simulink library "allblocks_alteradspbuilder2"  (Simulink 7.6)
(part 3 of 4)

      mask Help: helpview(char(com.altera.dspbuilder.simulation.Cache.getBlockTemplate('BlockFactory', 'com.altera.dspbuilder.blockset.arithmetic.SumOfProducts').getHelpFile))
      mask StyleString: popup(Signed Integer|Unsigned Integer|Signed Fractional|Unsigned Fractional),edit,edit,edit,edit,edit,edit,edit,edit,checkbox,edit,edit,edit,popup(Distributed Arithmetic|Dedicated Multiplier Circuitry|Auto),checkbox,checkbox
      mask CallbackString: |||||||||alt_dspbuilder_update_gui('BlockFactory', 'com.altera.dspbuilder.blockset.arithmetic.SumOfProducts', 'full_resolution', 9);||||||
      mask TabNameString: Main,Main,Main,Main,Main,Main,Main,Main,Main,Optional Port Sizing,Optional Port Sizing,Optional Port Sizing,Optional Port Sizing,Optional Ports and Settings,Optional Ports and Settings,Optional Ports and Settings
      mask Display:
      | port_label('input', 1, 'a0');
      | port_label('input', 2, 'a1');
      | port_label('input', 3, 'a2');
      | port_label('input', 4, 'a3');
      | port_label('output', 1, 'q(17:0)');
      | plot([0.9 0.75 0.85 0.75 0.9], [0.15 0.15 0.1 0.05 0.05])
  TestBench : S-Function  LoadFcn=|  FunctionName=sTestBench  Parameters=enable advancedMode modelSimGui maxDisplayErrors mismatchErrorLevel simdatafile  EnableBusSupport=off  mask(TestBench AlteraBlockset){enable=on, advancedMode=off, modelSimGui=off, maxDisplayErrors=10, mismatchErrorLevel=Error, simdatafile=}
      | alt_dspbuilder_load_block(gcb, 'BlockFactory', 'com.altera.dspbuilder.blockset.altlab.TestBench');
      | alt_dspbuilder_init_testbench
      mask prompts: enable "Enable test bench generation"; advancedMode "Use advanced mode"; modelSimGui "Launch ModelSim in Graphical mode"; maxDisplayErrors "Maximum number of errors to display"; mismatchErrorLevel "Error level for mismatches"
      mask help:
      | Controls automatic generation of a test bench. Enabling testbench generation may slow simulation as all input and output values are stored to a file.
      |
      | If the ModelSim executable (vsim.exe) is available on your path, you can load the testbench into ModelSim and compare the results with Simulink. You can optionally launch the ModelSim GUI to visually view the ModelSim simulation.
      mask init:
      | alt_dspbuilder_init_testbench('BlockFactory', 'com.altera.dspbuilder.blockset.altlab.TestBench', { enable advancedMode modelSimGui maxDisplayErrors mismatchErrorLevel simdatafile });
      settings: CopyFcn=alt_dspbuilder_add_block(gcb, 'BlockFactory', 'com.altera.dspbuilder.blockset.altlab.TestBench');  UndoDeleteFcn=alt_dspbuilder_add_block(gcb, 'BlockFactory', 'com.altera.dspbuilder.blockset.altlab.TestBench');  NameChangeFcn=alt_dspbuilder_block_renamed(gcb);
      settings: DeleteFcn=|
      | alt_dspbuilder_internal_remove_testbench(gcb)
      | 
      | com.altera.dspbuilder.simulation.Mask.delete(gcb);
      settings: PostSaveFcn=|
      | alt_dspbuilder_block_saved(gcb);
      | alt_dspbuilder_init_testbench
      settings: OpenFcn=|
      | com.altera.dspbuilder.simulation.Mask.simpleInit('BlockFactory', 'com.altera.dspbuilder.blockset.altlab.TestBench', bdroot(gcb), gcb);
      | alt_testbenchLaunch(gcb)
      mask Help: helpview(char(com.altera.dspbuilder.simulation.Cache.getBlockTemplate('BlockFactory', 'com.altera.dspbuilder.blockset.altlab.TestBench').getHelpFile))
      mask Display: fprintf('TestBench\non');
  True Dual-Port RAM : S-Function  LoadFcn=alt_dspbuilder_load_block(gcb, 'BlockFactory', 'com.altera.dspbuilder.blockset.storage.TrueDualRam');  FunctionName=sGeneric  Parameters=numwords BusType bwl bwr memory_type ram_type dont_care initialization init_file init_array register_outputs use_ena ClockPhase pipeline_display allowFloatingPointOverride logOutputs logFile  EnableBusSupport=off  mask(True Dual-Port RAM AlteraBlockset){numwords=16, BusType=Signed Integer, bwl=8, bwr=0, memory_type=AUTO, ram_type=TrueDualRAM, dont_care=off, initialization=Blank, init_file=input.hex, init_array=[0:1:15], register_outputs=off, use_ena=off, ClockPhase=1, pipeline_display=1, allowFloatingPointOverride=on, logOutputs=off, logFile=D:\\allblocks%5Falteradspbuilder2_True+Dual-Port+RAM%3A%3Aq%5Fa.fixedpointlog,D:\\allblocks%5Falteradspbuilder2_True+Dual-Port+RAM%3A%3Aq%5Fb.fixedpointlog,}
      mask prompts: numwords "Number Of Words"; BusType "Data Type"; bwl "[Number Of Bits].[]"; bwr "[].[Number Of Bits]"; memory_type "Memory Block Type"; ram_type "RAM type"; dont_care "Use DONT_CARE when reading from and writing to the same address"; init_file "Input HEX File"; init_array "MATLAB Array"; register_outputs "Register Output Ports"; use_ena "Use Enable Port (ena)"; ClockPhase "Clock Phase Selection"; pipeline_display "Number Of Pipeline Stages (Calculated)"; allowFloatingPointOverride "Allow Floating Point Override For This Block"
      mask help:
      | Maps data to embedded RAM in Altera devices. Two read and two write ports allow true dual access.
      |
      | The True Dual-Port RAM block accepts any type as Data input. The input port is registered, and the output port optionally registered.
      |
      | By default the contents of the RAM are pre-initialized to zero, but can be specified from an Intel-format hexadecimal (.hex) file, or from a MATLAB array.
      |
      | You can use the Quartus II software to generate a .hex file. Any specified ,hex file must be saved in your DSP Builder working directory.
      |
      | If used, the MATLAB array parameter must be a one dimensional MATLAB array with a length less than or equal to the number of words.
      | The array can be specified from the MATLAB work-space or directly in the MATLAB Array box.
      |
      | Note that the input address bus must be Unsigned, not all memory options are available for all device families, initialization is not possible for memory type M-RAM, and the clock enable (ena) bypasses any output register.
      mask init:
      | alt_dspbuilder_init('BlockFactory', 'com.altera.dspbuilder.blockset.storage.TrueDualRam', { numwords get_param(gcb, 'BusType') bwl bwr get_param(gcb, 'memory_type') ram_type dont_care get_param(gcb, 'initialization') init_file init_array register_outputs get_param(gcb, 'use_ena') ClockPhase pipeline_display allowFloatingPointOverride logOutputs logFile });
      settings: CopyFcn=alt_dspbuilder_add_block(gcb, 'BlockFactory', 'com.altera.dspbuilder.blockset.storage.TrueDualRam');  DeleteFcn=com.altera.dspbuilder.simulation.Mask.delete(gcb);  UndoDeleteFcn=alt_dspbuilder_add_block(gcb, 'BlockFactory', 'com.altera.dspbuilder.blockset.storage.TrueDualRam');  PostSaveFcn=alt_dspbuilder_block_saved(gcb);  NameChangeFcn=alt_dspbuilder_block_renamed(gcb);
      mask Help: helpview(char(com.altera.dspbuilder.simulation.Cache.getBlockTemplate('BlockFactory', 'com.altera.dspbuilder.blockset.storage.TrueDualRam').getHelpFile))
      mask StyleString: edit,popup(Inferred|Signed Integer|Unsigned Integer|Signed Fractional|Unsigned Fractional),edit,edit,popup(AUTO|M9K|M10K|M20K|M144K),popup(ROM|SingleRAM|DualRAM|TrueDualRAM),checkbox,popup(Blank|From HEX file|From MATLAB array),edit,edit,checkbox,checkbox,edit,edit,checkbox,checkbox,edit
      mask CallbackString: |alt_dspbuilder_update_gui('BlockFactory', 'com.altera.dspbuilder.blockset.storage.TrueDualRam', 'BusType', 1);|||alt_dspbuilder_update_gui('BlockFactory', 'com.altera.dspbuilder.blockset.storage.TrueDualRam', 'memory_type', 4);|||alt_dspbuilder_update_gui('BlockFactory', 'com.altera.dspbuilder.blockset.storage.TrueDualRam', 'initialization', 7);||||alt_dspbuilder_update_gui('BlockFactory', 'com.altera.dspbuilder.blockset.storage.TrueDualRam', 'use_ena', 11);|||||
      mask TabNameString: Main,Main,Main,Main,Main,Main,Main,Initialization,Initialization,Initialization,Registers and Enables,Registers and Enables,Registers and Enables,Registers and Enables,Registers and Enables,Registers and Enables,Registers and Enables
      mask Display:
      | port_label('input', 1, 'data_a(7:0)');
      | port_label('input', 2, 'addr_a(3:0)');
      | port_label('input', 3, 'wren_a');
      | port_label('input', 4, 'data_b(7:0)');
      | port_label('input', 5, 'addr_b(3:0)');
      | port_label('input', 6, 'wren_b');
      | port_label('output', 1, 'q_a');
      | port_label('output', 2, 'q_b');
      | fprintf('True DPRAM\n(%d x %d)' , 16, 8);
  Tsamp : S-Function  LoadFcn=alt_dspbuilder_load_block(gcb, 'BlockFactory', 'com.altera.dspbuilder.blockset.RateChange.Tsamp');  FunctionName=sGeneric  Parameters=SpecifyClock clock  EnableBusSupport=off  mask(Time Set AlteraBlockset){SpecifyClock=off, clock=Clock}
      mask prompts: SpecifyClock "Specify Clock"; clock "Clock Name"
      mask help:
      | Sets the clock domain inherited by all downstream blocks.
      |
      | When you use the Tsamp block, you must select a variable step solver in the Simulink configuration parameters. Unless the downstream clock is an exact, slower multiple of the upstream clock, the simulation results may not match ModelSim; in this case it is better to use a Multi-Rate DFF block.
      mask init:
      | alt_dspbuilder_init('BlockFactory', 'com.altera.dspbuilder.blockset.RateChange.Tsamp', { get_param(gcb, 'SpecifyClock') clock });
      settings: CopyFcn=alt_dspbuilder_add_block(gcb, 'BlockFactory', 'com.altera.dspbuilder.blockset.RateChange.Tsamp');  DeleteFcn=com.altera.dspbuilder.simulation.Mask.delete(gcb);  UndoDeleteFcn=alt_dspbuilder_add_block(gcb, 'BlockFactory', 'com.altera.dspbuilder.blockset.RateChange.Tsamp');  PostSaveFcn=alt_dspbuilder_block_saved(gcb);  NameChangeFcn=alt_dspbuilder_block_renamed(gcb);
      mask Help: helpview(char(com.altera.dspbuilder.simulation.Cache.getBlockTemplate('BlockFactory', 'com.altera.dspbuilder.blockset.RateChange.Tsamp').getHelpFile))
      mask CallbackString: alt_dspbuilder_update_gui('BlockFactory', 'com.altera.dspbuilder.blockset.RateChange.Tsamp', 'SpecifyClock', 0);|
      mask Display:
      | plot([0 2 18 20],[5 10 10 5]);
      | disp('INFER');
  Up Sampling : S-Function  LoadFcn=alt_dspbuilder_load_block(gcb, 'BlockFactory', 'com.altera.dspbuilder.blockset.storage.UpSampling');  FunctionName=sGeneric  Parameters=rate allowFloatingPointOverride logOutputs logFile  EnableBusSupport=off  mask(Up Sampling AlteraBlockset){rate=100, allowFloatingPointOverride=on, logOutputs=off, logFile=D:\\allblocks%5Falteradspbuilder2_Up+Sampling.fixedpointlog}
      mask prompts: rate "Up-sampling rate"; allowFloatingPointOverride "Allow Floating Point Override For This Block"
      mask help:
      | Increases the output sample rate from the input sample rate.
      | The output data is sampled every N cycles where N is equal to the up sampling rate.
      | The output holds this value for 1 cycle, then for the next N-1 cycles the output is zero.
      mask init:
      | alt_dspbuilder_init('BlockFactory', 'com.altera.dspbuilder.blockset.storage.UpSampling', { rate allowFloatingPointOverride logOutputs logFile });
      settings: CopyFcn=alt_dspbuilder_add_block(gcb, 'BlockFactory', 'com.altera.dspbuilder.blockset.storage.UpSampling');  DeleteFcn=com.altera.dspbuilder.simulation.Mask.delete(gcb);  UndoDeleteFcn=alt_dspbuilder_add_block(gcb, 'BlockFactory', 'com.altera.dspbuilder.blockset.storage.UpSampling');  PostSaveFcn=alt_dspbuilder_block_saved(gcb);  NameChangeFcn=alt_dspbuilder_block_renamed(gcb);
      mask Help: helpview(char(com.altera.dspbuilder.simulation.Cache.getBlockTemplate('BlockFactory', 'com.altera.dspbuilder.blockset.storage.UpSampling').getHelpFile))
      mask Display:
      | port_label('input', 1, 'd');
      | port_label('output', 1, 'q');
      | disp('x{100}','texmode','on');
  VCC : S-Function  LoadFcn=alt_dspbuilder_load_block(gcb, 'BlockFactory', 'com.altera.dspbuilder.blockset.iobus.VCC');  FunctionName=sGeneric  Parameters=SpecifyClock  EnableBusSupport=off  mask(VCC AlteraBlockset){SpecifyClock=off, clock=}
      mask prompts: SpecifyClock "Specify Clock"
      mask help: Outputs a single bit constant value of 1.
      mask init:
      | alt_dspbuilder_init('BlockFactory', 'com.altera.dspbuilder.blockset.iobus.VCC', { get_param(gcb, 'SpecifyClock') clock });
      settings: CopyFcn=alt_dspbuilder_add_block(gcb, 'BlockFactory', 'com.altera.dspbuilder.blockset.iobus.VCC');  DeleteFcn=com.altera.dspbuilder.simulation.Mask.delete(gcb);  UndoDeleteFcn=alt_dspbuilder_add_block(gcb, 'BlockFactory', 'com.altera.dspbuilder.blockset.iobus.VCC');  PostSaveFcn=alt_dspbuilder_block_saved(gcb);  NameChangeFcn=alt_dspbuilder_block_renamed(gcb);
      mask Help: helpview(char(com.altera.dspbuilder.simulation.Cache.getBlockTemplate('BlockFactory', 'com.altera.dspbuilder.blockset.iobus.VCC').getHelpFile))
      mask CallbackString: alt_dspbuilder_update_gui('BlockFactory', 'com.altera.dspbuilder.blockset.iobus.VCC', 'SpecifyClock', 0);|
      mask Display:
      | plot([1 0 0 1], [1 1 0 0])
      | disp('1');
  VCD Sink : S-Function  LoadFcn=alt_dspbuilder_load_block(gcb, 'BlockFactory', 'com.altera.dspbuilder.blockset.altlab.VCDSink');  InitFcn=alt_dspbuilder_internal_init_altlab_flow;  FunctionName=sGeneric  Parameters=inNames inBwls inBwrs inTypes inDelayed outNames outBwls outBwrs outTypes Inputs TextFilePath resetNames resetTypes resetLengths entityName  EnableBusSupport=off  mask(VCD Sink AlteraBlockset){inNames=Port1 Port2 Port3, inBwls=0 0 0, inBwrs=0 0 0, inTypes=i i i, inDelayed=1 1 1, outNames=, outBwls=, outBwrs=, outTypes=, Inputs=3, TextFilePath=, resetNames=, resetTypes=, resetLengths=, entityName=}
      mask prompts: Inputs "Number Of Inputs"; resetNames "array_clocks"; resetTypes "array_clocks"; resetLengths "array_clocks"
      mask help:
      | Exports Simulink signals to a third-party waveform viewer. The VCD Sink block generates a value change dump (.vcd) file named <block name>.vcd which can be read by the third-party waveform viewer. It also generates a Tcl script named <block name>_vcd.tcl which converts VCD files into ModelSim wave log format (.wlf) files, and launches the ModelSim waveform viewer.
      |
      | Step 1: Add the VCDSink block to your Simulink model.
      | Step 2: Connect the Simulink signals you want to display to the VCDSink block.
      | Step 3: Run the Simulink simulation.
      | Step 4: If you are using ModelSim simulator to view waveforms, run the script <block name>_vcd.tcl to convert the VCD file to a ModelSim WLF file. If using other tools, read the VCD file in the third-party waveform viewer directly.
      |
      | The VCDSink block does not have any hardware representation and therefore does not appear in the VHDL RTL representation created by the Signal Compiler block.
      mask init:
      | alt_dspbuilder_internal_VCD_sink_init('BlockFactory', 'com.altera.dspbuilder.blockset.altlab.VCDSink', { inNames inBwls inBwrs inTypes inDelayed outNames outBwls outBwrs outTypes Inputs TextFilePath resetNames resetTypes resetLengths entityName });
      settings: CopyFcn=alt_dspbuilder_add_block(gcb, 'BlockFactory', 'com.altera.dspbuilder.blockset.altlab.VCDSink');  DeleteFcn=com.altera.dspbuilder.simulation.Mask.delete(gcb);  UndoDeleteFcn=alt_dspbuilder_add_block(gcb, 'BlockFactory', 'com.altera.dspbuilder.blockset.altlab.VCDSink');  PostSaveFcn=alt_dspbuilder_block_saved(gcb);  NameChangeFcn=alt_dspbuilder_block_renamed(gcb);
      mask Help: helpview(char(com.altera.dspbuilder.simulation.Cache.getBlockTemplate('BlockFactory', 'com.altera.dspbuilder.blockset.altlab.VCDSink').getHelpFile))
      mask Display:
      | port_label('input', 1, 'Port1');
      | port_label('input', 2, 'Port2');
      | port_label('input', 3, 'Port3');
      | plot([-20],[0]);
      | plot([30],[30]);
      | plot([ 30 35 45 50 70 75 85 90 100 105 110 ],[ 10  5  5 10 10  5 5  10 10  5  5 ]);
      | plot([ 30 35 45 50 70 75 85 90 100 105 110 ],[  5 10 10  5  5 10 10  5  5 10 10 ]);
      | disp('VCD File');
  Variable Precision DSP Block : S-Function  LoadFcn=alt_dspbuilder_load_block(gcb, 'BlockFactory', 'com.altera.dspbuilder.blockset.arithmetic.VariablePrecisionDSPBlock');  FunctionName=sGeneric  Parameters=complex_model_delayed model_delayed device_family wysiwyg_device_family used_mode_stratix used_mode_arria in_25x18_complex_mode in_18x18plus36_mode in_other_modes number_of_mults clock_ena_inputs async_clear_inputs or_aclr_inputs bus_type bwl_A bwr_A width_A chain_width reg_inputs_A A_inputs_reg_ena bwl_B bwr_B width_B reg_inputs_B B_inputs_reg_ena bwl_joint_A_B bwr_joint_A_B reg_joint_A_B_input A_B_input_reg_ena bwl_A_complex bwr_A_complex reg_complex_A A_complex_inputs_reg_ena bwl_B_complex bwr_B_complex reg_complex_B B_complex_inputs_reg_ena all_inputs_registered no_input_registered all_inputs_share_same_clocks full_resolution bwl_out bwr_out bwl_out_complex bwr_out_complex bwl_18x18_mult bwr_18x18_mult bwl_out_18x18plus36 bwr_out_18x18plus36 bwl_preadder bwr_preadder bwl_out_other_modes bwr_out_other_modes bwr_out_full bwr_out_full_eval bwr_out_final bwl_out_full bwl_out_final output_lsb_final reg_output output_reg_ena systolic_regs_available enable_systolic_regs systolic_regs_used enable_input_pipeline_reg input_pipeline_reg_used input_pipeline_reg_ena basic_struct_ok_for_input_scan input_scan_available enable_input_scan input_scan_used use_scanin_input use_scanout_output input_scan_delay_regs_available enable_input_scan_delay_regs input_scan_delay_regs_used input_scan_delay_ay_reg_used basic_struct_ok_for_coef_rom coef_rom_available enable_coef_rom coef_rom_used basic_struct_ok_for_preadder preadder_available enable_preadder preadder_used preadder_direction square_mode_available enable_square_mode square_mode_used upper_limit_9bit upper_limit_18bit upper_limit_27bit in_9x9_mode in_18x18_modes in_27x27_modes in_36x18_modes in_36x36_mode A_inputs_exist B_inputs_exist C_inputs_exist coef_sel_inputs_exist mult1_adder_available mult1_direction mult3_adder_available mult3_direction chainout_adder_available use_chainout_input chainout_input_used use_chainout_output chainout_output_used accum_available enable_accum accum_used double_accum_available enable_double_accum double_accum_used negate_available mult_add_operation rounding_constant_available use_rounding_constant rounding_constant_used constant_value bwl_C bwr_C bwl_coef bwr_coef mult0_coeffs mult1_coeffs mult2_coeffs mult3_coeffs reg_mult1_op_control enable_addnsub1_pipeline_reg addnsub1_pipeline_reg_used reg_mult3_op_control reg_accum_control enable_accum_pipeline_reg accum_pipeline_reg_used reg_negate_control enable_negate_pipeline_reg negate_pipeline_reg_used any_control_input_exist control_regs_ena control_pipeline_regs_ena ena0_used ena1_used ena2_used  EnableBusSupport=off  mask(StratixV ArriaV and CycloneV Variable Precision DSP Block AlteraBlockset){complex_model_delayed=0, model_delayed=0, device_family=Stratix V, wysiwyg_device_family=stratixv, used_mode_stratix=Other Modes, used_mode_arria=Other Modes, in_25x18_complex_mode=0, in_18x18plus36_mode=0, in_other_modes=1, number_of_mults=1, clock_ena_inputs=off, async_clear_inputs=off, or_aclr_inputs=on, bus_type=Unsigned Integer, bwl_A=8, bwr_A=0, width_A=8, chain_width=64, reg_inputs_A=on, A_inputs_reg_ena=ENABLE 0, bwl_B=8, bwr_B=0, width_B=8, reg_inputs_B=on, B_inputs_reg_ena=ENABLE 0, bwl_joint_A_B=8, bwr_joint_A_B=0, reg_joint_A_B_input=on, A_B_input_reg_ena=ENABLE 0, bwl_A_complex=8, bwr_A_complex=8, reg_complex_A=on, A_complex_inputs_reg_ena=ENABLE 0, bwl_B_complex=8, bwr_B_complex=8, reg_complex_B=on, B_complex_inputs_reg_ena=ENABLE 0, all_inputs_registered=1, no_input_registered=0, all_inputs_share_same_clocks=1, full_resolution=off, bwl_out=16, bwr_out=0, bwl_out_complex=17, bwr_out_complex=16, bwl_18x18_mult=16, bwr_18x18_mult=0, bwl_out_18x18plus36=17, bwr_out_18x18plus36=0, bwl_preadder=9, bwr_preadder=0, bwl_out_other_modes=16, bwr_out_other_modes=0, bwr_out_full=0, bwr_out_full_eval=0, bwr_out_final=0, bwl_out_full=16, bwl_out_final=16, output_lsb_final=0, reg_output=on, output_reg_ena=ENABLE 0, systolic_regs_available=0, enable_systolic_regs=off, systolic_regs_used=0, enable_input_pipeline_reg=off, input_pipeline_reg_used=0, input_pipeline_reg_ena=ENABLE 0, basic_struct_ok_for_input_scan=1, input_scan_available=1, enable_input_scan=off, input_scan_used=0, use_scanin_input=off, use_scanout_output=off, input_scan_delay_regs_available=0, enable_input_scan_delay_regs=off, input_scan_delay_regs_used=0, input_scan_delay_ay_reg_used=0, basic_struct_ok_for_coef_rom=1, coef_rom_available=1, enable_coef_rom=off, coef_rom_used=0, basic_struct_ok_for_preadder=1, preadder_available=0, enable_preadder=off, preadder_used=0, preadder_direction=ADD, square_mode_available=0, enable_square_mode=off, square_mode_used=0, upper_limit_9bit=9, upper_limit_18bit=18, upper_limit_27bit=27, in_9x9_mode=1, in_18x18_modes=1, in_27x27_modes=0, in_36x18_modes=0, in_36x36_mode=0, A_inputs_exist=1, B_inputs_exist=1, C_inputs_exist=0, coef_sel_inputs_exist=0, mult1_adder_available=0, mult1_direction=ADD, mult3_adder_available=0, mult3_direction=ADD, chainout_adder_available=0, use_chainout_input=off, chainout_input_used=0, use_chainout_output=off, chainout_output_used=0, accum_available=0, enable_accum=off, accum_used=0, double_accum_available=0, enable_double_accum=off, double_accum_used=0, negate_available=0, mult_add_operation=ADD, rounding_constant_available=0, use_rounding_constant=off, rounding_constant_used=0, constant_value=0, bwl_C=8, bwr_C=0, bwl_coef=18, bwr_coef=0, mult0_coeffs=[0, 0, 0, 0, 0, 0, 0, 0], mult1_coeffs=[0, 0, 0, 0, 0, 0, 0, 0], mult2_coeffs=[0, 0, 0, 0, 0, 0, 0, 0], mult3_coeffs=[0, 0, 0, 0, 0, 0, 0, 0], reg_mult1_op_control=off, enable_addnsub1_pipeline_reg=off, addnsub1_pipeline_reg_used=0, reg_mult3_op_control=off, reg_accum_control=off, enable_accum_pipeline_reg=off, accum_pipeline_reg_used=0, reg_negate_control=off, enable_negate_pipeline_reg=off, negate_pipeline_reg_used=0, any_control_input_exist=0, control_regs_ena=ENABLE 0, control_pipeline_regs_ena=ENABLE 0, ena0_used=1, ena1_used=0, ena2_used=0}
      mask prompts: complex_model_delayed "Whether there are any registers in Complex Model"; model_delayed "Whether there are any registers in NON Complex Model"; device_family "Device Family"; used_mode_stratix "Use Block for"; used_mode_arria "Use Block for"; in_25x18_complex_mode "Is in 25x18 Complex mode"; in_18x18plus36_mode "Is in 18x18+36 mode"; in_other_modes "In Other than Complex and 18x18+36 Modes"; number_of_mults "Number of Multipliers (1-4, where 3,4 are Available for Stratix V Only)"; clock_ena_inputs "Use Enable Inputs (ena0/1/2)"; async_clear_inputs "Use Asynchronous Clear Inputs (aclr0/1)"; or_aclr_inputs "'OR' Asynchronous Clear Inputs with Global Aclr"; bus_type "Bus Type"; bwl_A "'a' Input(s) [Number of Bits].[]"; bwr_A "'a' Input(s) [].[Number of Bits]"; width_A "A Overall Width"; chain_width "Width is 64 for all modes, except systolic mode, where it is 44"; reg_inputs_A "Register 'a' Input(s)"; A_inputs_reg_ena "Enable for 'a' Input(s) Register"; bwl_B "'b' Input(s) [Number of Bits].[]"; bwr_B "'b' Input(s) [].[Number of Bits]"; width_B "B Overall Width"; reg_inputs_B "Register 'b' Input(s)"; B_inputs_reg_ena "Enable for 'b' Input(s) Register"; bwl_joint_A_B "Joint 'ab' Input [Number of Bits].[]"; bwr_joint_A_B "Joint 'ab' Input [].[Number of Bits]"; reg_joint_A_B_input "Register Joint 'ab' Input"; A_B_input_reg_ena "Enable for Joint 'ab' Input Register"; bwl_A_complex "'a' Real/Imaginary Input [Number of Bits].[]"; bwr_A_complex "'a' Real/Imaginary Input [].[Number of Bits]"; reg_complex_A "Register 'a' Real/Imaginary Inputs"; A_complex_inputs_reg_ena "Enable for 'a' Real/Imaginary Inputs Register"; bwl_B_complex "'b' Real/Imaginary Input [Number of Bits].[]"; bwr_B_complex "'b' Real/Imaginary Input [].[Number of Bits]"; reg_complex_B "Register 'b' Real/Imaginary Inputs"; B_complex_inputs_reg_ena "Enable for 'b' Real/Imaginary Inputs Register"; all_inputs_registered "All Inputs Registered"; no_input_registered "None of Inputs is Registered"; all_inputs_share_same_clocks "All Inputs Share the Same Clock Settings"; full_resolution "Enable Output Full Resolution"; bwl_out "Output [Number of Bits].[]"; bwr_out "Output [].[Number of Bits]"; bwl_out_complex "Calculated full output bwl in complex mode"; bwr_out_complex "Calculated full output bwr in complex mode"; bwl_18x18_mult "bwl for multiplication in 18x18+36 mode"; bwr_18x18_mult "bwr for multiplication in 18x18+36 mode"; bwl_out_18x18plus36 "bwl for output in 18x18+36 mode"; bwr_out_18x18plus36 "bwr for output in 18x18+36 mode calculation"; bwl_preadder "bwl for PreAdder result in Other Modes"; bwr_preadder "bwl for PreAdder result in Other Modes"; bwr_out_full "Full resolution output bwr"; bwr_out_full_eval "Full resolution output bwr"; bwr_out_final "Final output bwr"; bwl_out_full "Full resolution output bwl"; bwl_out_final "Final output bwl"; output_lsb_final "Number of bwr bits to remove"; reg_output "Register Output"; output_reg_ena "Enable for Ouput Register"; systolic_regs_available "Whether Systolic Registers can be enabled"; enable_systolic_regs "Enable Systolic Registers"; systolic_regs_used "Whether Systolic registers ARE actually used"; enable_input_pipeline_reg "Enable Data Inputs Pipeline Register"; input_pipeline_reg_ena "Enable for Pipeline Registers (including control pipeline registers if used)"; basic_struct_ok_for_input_scan "Basic Structure and Primary Data Widths OK for Input Scan Chain"; input_scan_available "Whether Input Scan Chain IS Available"; enable_input_scan "Enable Input Scan Chain"; input_scan_used "Whether Input Scan Chain SHOULD be Used"; use_scanin_input "Use 'scanin' Input"; use_scanout_output "Use 'scanout' Output"; input_scan_delay_regs_available "Whether Input Scan Delay Registers CAN be Used"; enable_input_scan_delay_regs "Enable Input Scan Chain Delay Registers"; input_scan_delay_regs_used "Whether Input Scan Delay Registers SHOULD be Used"; input_scan_delay_ay_reg_used "Whether Input Scan Delay Register on AY line should be Used"; basic_struct_ok_for_coef_rom "Basic Structure and Primary Data Widths OK for Coefficient ROM"; coef_rom_available "Whether Coefficient ROM CAN be Enabled"; enable_coef_rom "Enable Coefficient ROM"; coef_rom_used "Whether Coefficient ROM SHOULD be Enabled"; basic_struct_ok_for_preadder "Basic Structure and Primary Data Widths OK for PreAdder"; preadder_available "Whether Pre Adder feature CAN be enabled for the block"; enable_preadder "Enable PreAdder"; preadder_used "Whether Pre Adder feature SHOULD be enabled for the block"; preadder_direction "PreAdder Direction"; square_mode_available "Whether Pre Adder Square mode CAN be used"; enable_square_mode "Connect Same PreAdder Output to Both Multiplier Inputs"; square_mode_used "Whether Pre Adder Square mode SHOULD be used"; upper_limit_9bit "Upper limit for data bit width to be in 9bit mode"; upper_limit_18bit "Upper limit for data bit width to be in 18bit mode"; upper_limit_27bit "Upper limit for data bit width to be in 27bit mode"; in_9x9_mode "Whether the block is in 9x9 mode"; in_18x18_modes "Whether the block is in any of possible 18x18 modes"; in_27x27_modes "Whether the block is in any of possible 27x27 modes"; in_36x18_modes "Whether the block is in any of possible 36x18 modes (for Stratix V only)"; in_36x36_mode "Whether the block is in 36x36 mode (for Stratix V only)"; A_inputs_exist "A Inputs (except A1) Exist"; B_inputs_exist "B Inputs Exist"; C_inputs_exist "C Inputs Exist"; coef_sel_inputs_exist "Coef Sel Inputs Exist"; mult1_adder_available "Whether block is configured to use Adder after first Mults pair"; mult1_direction "Output Operation on First Multiplier Pair"; mult3_adder_available "Whether block is configured to use Adder after second Mults pair"; mult3_direction "Output Operation on Second Multiplier Pair"; chainout_adder_available "Whether chainout adder CAN be used for the block"; use_chainout_input "Use Chainout Adder Input (chainin)"; chainout_input_used "Whether ChainOut Input is USED for the block"; use_chainout_output "Use Chainout Adder Output (chainout)"; chainout_output_used "Whether ChainOut Output is USED for the block"; accum_available "Whether accumulation feature CAN be enabled for the block"; enable_accum "Enable Accumulation (dynamically controlled if On)"; accum_used "Whether accumulation feature SHOULD be enabled for the block"; double_accum_available "Whether double accumulation register CAN be enabled for the block"; enable_double_accum "Enable Double Accumulation Register"; double_accum_used "Whether double accumulation register SHOULD be enabled for the block"; negate_available "Whether Negate Control is available"; mult_add_operation "Operation on Multiplier-Adder Output"; rounding_constant_available "Whether Rounding Constant feature CAN be used"; use_rounding_constant "Use Rounding Constant"; rounding_constant_used "Whether Rounding Constant feature SHOULD be used"; constant_value "Rounding Constant Value"; bwl_C "'c' Input(s) [Number of Bits].[]"; bwr_C "'c' Input(s) [].[Number of Bits]"; bwl_coef "Coefficient Values [Number of Bits].[]"; bwr_coef "Coefficient Values [].[Number of Bits]"; mult0_coeffs "Coefficients for First Multiplier"; mult1_coeffs "Coefficients for Second Multiplier"; mult2_coeffs "Coefficients for Third Multiplier"; mult3_coeffs "Coefficients for Forth Multiplier"; reg_mult1_op_control "Register Control Input for First Multiplier Pair Output Operation (addnsub1)"; enable_addnsub1_pipeline_reg "Enable Pipeline Register for 'addnsub1'"; addnsub1_pipeline_reg_used "Whether addnsub1 pipeline register actually should be used"; reg_mult3_op_control "Register Control Input for Second Multiplier Pair Output Operation (addnsub3)"; reg_accum_control "Register Control Input for Accumulation (accum)"; enable_accum_pipeline_reg "Enable Pipeline Register for 'accum'"; accum_pipeline_reg_used "Whether accum pipeline register actually should be used"; reg_negate_control "Register Control Input for Multiplier-Adder Output Operation (negate)"; enable_negate_pipeline_reg "Enable Pipeline Register for 'negate'"; negate_pipeline_reg_used "Whether negate pipeline register actually should be used"; any_control_input_exist "Whether any of control inputs exists."; control_regs_ena "Enable for Control Input(s) Register"; control_pipeline_regs_ena "Enable for Control Inputs(s) Pipeline Register"; ena0_used "Enable0 is actually used"; ena1_used "Enable1 is actually used"; ena2_used "Enable2 is actually used"
      mask help:
      | Variable Precision DSP block exposes most of the features of 28 nm DSP Block available on Stratix V, Arria V and Cyclone V devices.
      |
      | The block accepts up to 4 pairs of multiplier inputs. The results of multiplication are being summed or subtracted based on block configuration.
      | The example equation for two multipliers is: +/-(A0 * B0) + (A1 * B1)
      |
      | The accumulation can be controlled through a special control input. Several DSP blocks can be chained together by enabling chainout adder (chainin/chainout ports).
      | Simple rounding operation can be performed on the final result using the rounding constant value.
      |
      | Pre Adder and Coefficient ROM blocks can be enabled to feed multipliers. An expression for one multiplier being feed by Pre Adder and Coefficient ROM is: (B0 +/- A0) * ROM[coef_sel0]
      |
      | Please refer to DSP Builder Help or the Quartus II altera_mult_add Megafunction documentation for more information.
      |
      | For Stratix V family only, the block can be configured to do complex multiplication.
      |
      | NOTE: Please press 'Apply' after changes to parameter values to refresh the GUI and activate parameter value checks. Changes which affect the list of ports may require several GUI refreshes.
      mask init:
      | alt_dspbuilder_init('BlockFactory', 'com.altera.dspbuilder.blockset.arithmetic.VariablePrecisionDSPBlock', { complex_model_delayed model_delayed get_param(gcb, 'device_family') wysiwyg_device_family get_param(gcb, 'used_mode_stratix') get_param(gcb, 'used_mode_arria') get_param(gcb, 'in_25x18_complex_mode') get_param(gcb, 'in_18x18plus36_mode') get_param(gcb, 'in_other_modes') get_param(gcb, 'number_of_mults') get_param(gcb, 'clock_ena_inputs') get_param(gcb, 'async_clear_inputs') get_param(gcb, 'or_aclr_inputs') get_param(gcb, 'bus_type') bwl_A bwr_A width_A chain_width get_param(gcb, 'reg_inputs_A') A_inputs_reg_ena bwl_B bwr_B width_B get_param(gcb, 'reg_inputs_B') B_inputs_reg_ena bwl_joint_A_B bwr_joint_A_B get_param(gcb, 'reg_joint_A_B_input') A_B_input_reg_ena bwl_A_complex bwr_A_complex get_param(gcb, 'reg_complex_A') A_complex_inputs_reg_ena bwl_B_complex bwr_B_complex get_param(gcb, 'reg_complex_B') B_complex_inputs_reg_ena get_param(gcb, 'all_inputs_registered') get_param(gcb, 'no_input_registered') get_param(gcb, 'all_inputs_share_same_clocks') get_param(gcb, 'full_resolution') bwl_out bwr_out bwl_out_complex bwr_out_complex bwl_18x18_mult bwr_18x18_mult bwl_out_18x18plus36 bwr_out_18x18plus36 bwl_preadder bwr_preadder bwl_out_other_modes bwr_out_other_modes bwr_out_full bwr_out_full_eval bwr_out_final bwl_out_full bwl_out_final output_lsb_final get_param(gcb, 'reg_output') output_reg_ena get_param(gcb, 'systolic_regs_available') get_param(gcb, 'enable_systolic_regs') get_param(gcb, 'systolic_regs_used') get_param(gcb, 'enable_input_pipeline_reg') get_param(gcb, 'input_pipeline_reg_used') input_pipeline_reg_ena get_param(gcb, 'basic_struct_ok_for_input_scan') get_param(gcb, 'input_scan_available') get_param(gcb, 'enable_input_scan') get_param(gcb, 'input_scan_used') get_param(gcb, 'use_scanin_input') get_param(gcb, 'use_scanout_output') get_param(gcb, 'input_scan_delay_regs_available') get_param(gcb, 'enable_input_scan_delay_regs') get_param(gcb, 'input_scan_delay_regs_used') get_param(gcb, 'input_scan_delay_ay_reg_used') get_param(gcb, 'basic_struct_ok_for_coef_rom') get_param(gcb, 'coef_rom_available') get_param(gcb, 'enable_coef_rom') get_param(gcb, 'coef_rom_used') get_param(gcb, 'basic_struct_ok_for_preadder') get_param(gcb, 'preadder_available') get_param(gcb, 'enable_preadder') get_param(gcb, 'preadder_used') preadder_direction get_param(gcb, 'square_mode_available') get_param(gcb, 'enable_square_mode') get_param(gcb, 'square_mode_used') upper_limit_9bit get_param(gcb, 'upper_limit_18bit') get_param(gcb, 'upper_limit_27bit') get_param(gcb, 'in_9x9_mode') get_param(gcb, 'in_18x18_modes') get_param(gcb, 'in_27x27_modes') get_param(gcb, 'in_36x18_modes') get_param(gcb, 'in_36x36_mode') get_param(gcb, 'A_inputs_exist') get_param(gcb, 'B_inputs_exist') get_param(gcb, 'C_inputs_exist') get_param(gcb, 'coef_sel_inputs_exist') get_param(gcb, 'mult1_adder_available') get_param(gcb, 'mult1_direction') get_param(gcb, 'mult3_adder_available') get_param(gcb, 'mult3_direction') get_param(gcb, 'chainout_adder_available') get_param(gcb, 'use_chainout_input') get_param(gcb, 'chainout_input_used') get_param(gcb, 'use_chainout_output') get_param(gcb, 'chainout_output_used') get_param(gcb, 'accum_available') get_param(gcb, 'enable_accum') get_param(gcb, 'accum_used') get_param(gcb, 'double_accum_available') get_param(gcb, 'enable_double_accum') get_param(gcb, 'double_accum_used') get_param(gcb, 'negate_available') get_param(gcb, 'mult_add_operation') get_param(gcb, 'rounding_constant_available') get_param(gcb, 'use_rounding_constant') get_param(gcb, 'rounding_constant_used') constant_value bwl_C bwr_C bwl_coef bwr_coef mult0_coeffs mult1_coeffs mult2_coeffs mult3_coeffs get_param(gcb, 'reg_mult1_op_control') get_param(gcb, 'enable_addnsub1_pipeline_reg') addnsub1_pipeline_reg_used get_param(gcb, 'reg_mult3_op_control') get_param(gcb, 'reg_accum_control') get_param(gcb, 'enable_accum_pipeline_reg') accum_pipeline_reg_used get_param(gcb, 'reg_negate_control') get_param(gcb, 'enable_negate_pipeline_reg') negate_pipeline_reg_used any_control_input_exist get_param(gcb, 'control_regs_ena') get_param(gcb, 'control_pipeline_regs_ena') ena0_used ena1_used ena2_used });
      settings: CopyFcn=alt_dspbuilder_add_block(gcb, 'BlockFactory', 'com.altera.dspbuilder.blockset.arithmetic.VariablePrecisionDSPBlock');  DeleteFcn=com.altera.dspbuilder.simulation.Mask.delete(gcb);  UndoDeleteFcn=alt_dspbuilder_add_block(gcb, 'BlockFactory', 'com.altera.dspbuilder.blockset.arithmetic.VariablePrecisionDSPBlock');  PostSaveFcn=alt_dspbuilder_block_saved(gcb);  NameChangeFcn=alt_dspbuilder_block_renamed(gcb);
      mask Help: helpview(char(com.altera.dspbuilder.simulation.Cache.getBlockTemplate('BlockFactory', 'com.altera.dspbuilder.blockset.arithmetic.VariablePrecisionDSPBlock').getHelpFile))
      mask StyleString: edit,edit,popup(Stratix V|Arria V|Cyclone V),edit,popup(25x18 Complex Mode|18x18+36 Mode|Other Modes),popup(18x18+36 Mode|Other Modes),edit,edit,edit,popup(1|2|3|4),checkbox,checkbox,checkbox,popup(Signed Integer|Unsigned Integer|Signed Fractional|Unsigned Fractional),edit,edit,edit,edit,checkbox,popup(ENABLE 0|ENABLE 1|ENABLE 2),edit,edit,edit,checkbox,popup(ENABLE 0|ENABLE 1|ENABLE 2),edit,edit,checkbox,popup(ENABLE 0|ENABLE 1|ENABLE 2),edit,edit,checkbox,popup(ENABLE 0|ENABLE 1|ENABLE 2),edit,edit,checkbox,popup(ENABLE 0|ENABLE 1|ENABLE 2),edit,edit,edit,checkbox,edit,edit,edit,edit,edit,edit,edit,edit,edit,edit,edit,edit,edit,edit,edit,edit,edit,edit,checkbox,popup(ENABLE 0|ENABLE 1|ENABLE 2),edit,checkbox,edit,checkbox,edit,popup(ENABLE 0|ENABLE 1|ENABLE 2),edit,edit,checkbox,edit,checkbox,checkbox,edit,checkbox,edit,edit,edit,edit,checkbox,edit,edit,edit,checkbox,edit,popup(ADD|SUB),edit,checkbox,edit,edit,edit,edit,edit,edit,edit,edit,edit,edit,edit,edit,edit,edit,popup(ADD|SUB|VARIABLE),edit,popup(ADD|SUB|VARIABLE),edit,checkbox,edit,checkbox,edit,edit,checkbox,edit,edit,checkbox,edit,edit,popup(ADD|SUB|VARIABLE),edit,checkbox,edit,edit,edit,edit,edit,edit,edit,edit,edit,edit,checkbox,checkbox,edit,checkbox,checkbox,checkbox,edit,checkbox,checkbox,edit,edit,popup(ENABLE 0|ENABLE 1|ENABLE 2),popup(ENABLE 0|ENABLE 1|ENABLE 2),edit,edit,edit
      mask CallbackString: ||alt_dspbuilder_update_gui('BlockFactory', 'com.altera.dspbuilder.blockset.arithmetic.VariablePrecisionDSPBlock', 'device_family', 2);||alt_dspbuilder_update_gui('BlockFactory', 'com.altera.dspbuilder.blockset.arithmetic.VariablePrecisionDSPBlock', 'used_mode_stratix', 4);|alt_dspbuilder_update_gui('BlockFactory', 'com.altera.dspbuilder.blockset.arithmetic.VariablePrecisionDSPBlock', 'used_mode_arria', 5);|alt_dspbuilder_update_gui('BlockFactory', 'com.altera.dspbuilder.blockset.arithmetic.VariablePrecisionDSPBlock', 'in_25x18_complex_mode', 6);|alt_dspbuilder_update_gui('BlockFactory', 'com.altera.dspbuilder.blockset.arithmetic.VariablePrecisionDSPBlock', 'in_18x18plus36_mode', 7);|alt_dspbuilder_update_gui('BlockFactory', 'com.altera.dspbuilder.blockset.arithmetic.VariablePrecisionDSPBlock', 'in_other_modes', 8);|alt_dspbuilder_update_gui('BlockFactory', 'com.altera.dspbuilder.blockset.arithmetic.VariablePrecisionDSPBlock', 'number_of_mults', 9);|alt_dspbuilder_update_gui('BlockFactory', 'com.altera.dspbuilder.blockset.arithmetic.VariablePrecisionDSPBlock', 'clock_ena_inputs', 10);|alt_dspbuilder_update_gui('BlockFactory', 'com.altera.dspbuilder.blockset.arithmetic.VariablePrecisionDSPBlock', 'async_clear_inputs', 11);|alt_dspbuilder_update_gui('BlockFactory', 'com.altera.dspbuilder.blockset.arithmetic.VariablePrecisionDSPBlock', 'or_aclr_inputs', 12);|alt_dspbuilder_update_gui('BlockFactory', 'com.altera.dspbuilder.blockset.arithmetic.VariablePrecisionDSPBlock', 'bus_type', 13);|||||alt_dspbuilder_update_gui('BlockFactory', 'com.altera.dspbuilder.blockset.arithmetic.VariablePrecisionDSPBlock', 'reg_inputs_A', 18);|||||alt_dspbuilder_update_gui('BlockFactory', 'com.altera.dspbuilder.blockset.arithmetic.VariablePrecisionDSPBlock', 'reg_inputs_B', 23);||||alt_dspbuilder_update_gui('BlockFactory', 'com.altera.dspbuilder.blockset.arithmetic.VariablePrecisionDSPBlock', 'reg_joint_A_B_input', 27);||||alt_dspbuilder_update_gui('BlockFactory', 'com.altera.dspbuilder.blockset.arithmetic.VariablePrecisionDSPBlock', 'reg_complex_A', 31);||||alt_dspbuilder_update_gui('BlockFactory', 'com.altera.dspbuilder.blockset.arithmetic.VariablePrecisionDSPBlock', 'reg_complex_B', 35);||alt_dspbuilder_update_gui('BlockFactory', 'com.altera.dspbuilder.blockset.arithmetic.VariablePrecisionDSPBlock', 'all_inputs_registered', 37);|alt_dspbuilder_update_gui('BlockFactory', 'com.altera.dspbuilder.blockset.arithmetic.VariablePrecisionDSPBlock', 'no_input_registered', 38);|alt_dspbuilder_update_gui('BlockFactory', 'com.altera.dspbuilder.blockset.arithmetic.VariablePrecisionDSPBlock', 'all_inputs_share_same_clocks', 39);|alt_dspbuilder_update_gui('BlockFactory', 'com.altera.dspbuilder.blockset.arithmetic.VariablePrecisionDSPBlock', 'full_resolution', 40);|||||||||||||||||||alt_dspbuilder_update_gui('BlockFactory', 'com.altera.dspbuilder.blockset.arithmetic.VariablePrecisionDSPBlock', 'reg_output', 59);||alt_dspbuilder_update_gui('BlockFactory', 'com.altera.dspbuilder.blockset.arithmetic.VariablePrecisionDSPBlock', 'systolic_regs_available', 61);|alt_dspbuilder_update_gui('BlockFactory', 'com.altera.dspbuilder.blockset.arithmetic.VariablePrecisionDSPBlock', 'enable_systolic_regs', 62);|alt_dspbuilder_update_gui('BlockFactory', 'com.altera.dspbuilder.blockset.arithmetic.VariablePrecisionDSPBlock', 'systolic_regs_used', 63);|alt_dspbuilder_update_gui('BlockFactory', 'com.altera.dspbuilder.blockset.arithmetic.VariablePrecisionDSPBlock', 'enable_input_pipeline_reg', 64);|alt_dspbuilder_update_gui('BlockFactory', 'com.altera.dspbuilder.blockset.arithmetic.VariablePrecisionDSPBlock', 'input_pipeline_reg_used', 65);||alt_dspbuilder_update_gui('BlockFactory', 'com.altera.dspbuilder.blockset.arithmetic.VariablePrecisionDSPBlock', 'basic_struct_ok_for_input_scan', 67);|alt_dspbuilder_update_gui('BlockFactory', 'com.altera.dspbuilder.blockset.arithmetic.VariablePrecisionDSPBlock', 'input_scan_available', 68);|alt_dspbuilder_update_gui('BlockFactory', 'com.altera.dspbuilder.blockset.arithmetic.VariablePrecisionDSPBlock', 'enable_input_scan', 69);|alt_dspbuilder_update_gui('BlockFactory', 'com.altera.dspbuilder.blockset.arithmetic.VariablePrecisionDSPBlock', 'input_scan_used', 70);|alt_dspbuilder_update_gui('BlockFactory', 'com.altera.dspbuilder.blockset.arithmetic.VariablePrecisionDSPBlock', 'use_scanin_input', 71);|alt_dspbuilder_update_gui('BlockFactory', 'com.altera.dspbuilder.blockset.arithmetic.VariablePrecisionDSPBlock', 'use_scanout_output', 72);|alt_dspbuilder_update_gui('BlockFactory', 'com.altera.dspbuilder.blockset.arithmetic.VariablePrecisionDSPBlock', 'input_scan_delay_regs_available', 73);|alt_dspbuilder_update_gui('BlockFactory', 'com.altera.dspbuilder.blockset.arithmetic.VariablePrecisionDSPBlock', 'enable_input_scan_delay_regs', 74);|alt_dspbuilder_update_gui('BlockFactory', 'com.altera.dspbuilder.blockset.arithmetic.VariablePrecisionDSPBlock', 'input_scan_delay_regs_used', 75);|alt_dspbuilder_update_gui('BlockFactory', 'com.altera.dspbuilder.blockset.arithmetic.VariablePrecisionDSPBlock', 'input_scan_delay_ay_reg_used', 76);|alt_dspbuilder_update_gui('BlockFactory', 'com.altera.dspbuilder.blockset.arithmetic.VariablePrecisionDSPBlock', 'basic_struct_ok_for_coef_rom', 77);|alt_dspbuilder_update_gui('BlockFactory', 'com.altera.dspbuilder.blockset.arithmetic.VariablePrecisionDSPBlock', 'coef_rom_available', 78);|alt_dspbuilder_update_gui('BlockFactory', 'com.altera.dspbuilder.blockset.arithmetic.VariablePrecisionDSPBlock', 'enable_coef_rom', 79);|alt_dspbuilder_update_gui('BlockFactory', 'com.altera.dspbuilder.blockset.arithmetic.VariablePrecisionDSPBlock', 'coef_rom_used', 80);|alt_dspbuilder_update_gui('BlockFactory', 'com.altera.dspbuilder.blockset.arithmetic.VariablePrecisionDSPBlock', 'basic_struct_ok_for_preadder', 81);|alt_dspbuilder_update_gui('BlockFactory', 'com.altera.dspbuilder.blockset.arithmetic.VariablePrecisionDSPBlock', 'preadder_available', 82);|alt_dspbuilder_update_gui('BlockFactory', 'com.altera.dspbuilder.blockset.arithmetic.VariablePrecisionDSPBlock', 'enable_preadder', 83);|alt_dspbuilder_update_gui('BlockFactory', 'com.altera.dspbuilder.blockset.arithmetic.VariablePrecisionDSPBlock', 'preadder_used', 84);||alt_dspbuilder_update_gui('BlockFactory', 'com.altera.dspbuilder.blockset.arithmetic.VariablePrecisionDSPBlock', 'square_mode_available', 86);|alt_dspbuilder_update_gui('BlockFactory', 'com.altera.dspbuilder.blockset.arithmetic.VariablePrecisionDSPBlock', 'enable_square_mode', 87);|alt_dspbuilder_update_gui('BlockFactory', 'com.altera.dspbuilder.blockset.arithmetic.VariablePrecisionDSPBlock', 'square_mode_used', 88);||alt_dspbuilder_update_gui('BlockFactory', 'com.altera.dspbuilder.blockset.arithmetic.VariablePrecisionDSPBlock', 'upper_limit_18bit', 90);|alt_dspbuilder_update_gui('BlockFactory', 'com.altera.dspbuilder.blockset.arithmetic.VariablePrecisionDSPBlock', 'upper_limit_27bit', 91);|alt_dspbuilder_update_gui('BlockFactory', 'com.altera.dspbuilder.blockset.arithmetic.VariablePrecisionDSPBlock', 'in_9x9_mode', 92);|alt_dspbuilder_update_gui('BlockFactory', 'com.altera.dspbuilder.blockset.arithmetic.VariablePrecisionDSPBlock', 'in_18x18_modes', 93);|alt_dspbuilder_update_gui('BlockFactory', 'com.altera.dspbuilder.blockset.arithmetic.VariablePrecisionDSPBlock', 'in_27x27_modes', 94);|alt_dspbuilder_update_gui('BlockFactory', 'com.altera.dspbuilder.blockset.arithmetic.VariablePrecisionDSPBlock', 'in_36x18_modes', 95);|alt_dspbuilder_update_gui('BlockFactory', 'com.altera.dspbuilder.blockset.arithmetic.VariablePrecisionDSPBlock', 'in_36x36_mode', 96);|alt_dspbuilder_update_gui('BlockFactory', 'com.altera.dspbuilder.blockset.arithmetic.VariablePrecisionDSPBlock', 'A_inputs_exist', 97);|alt_dspbuilder_update_gui('BlockFactory', 'com.altera.dspbuilder.blockset.arithmetic.VariablePrecisionDSPBlock', 'B_inputs_exist', 98);|alt_dspbuilder_update_gui('BlockFactory', 'com.altera.dspbuilder.blockset.arithmetic.VariablePrecisionDSPBlock', 'C_inputs_exist', 99);|alt_dspbuilder_update_gui('BlockFactory', 'com.altera.dspbuilder.blockset.arithmetic.VariablePrecisionDSPBlock', 'coef_sel_inputs_exist', 100);|alt_dspbuilder_update_gui('BlockFactory', 'com.altera.dspbuilder.blockset.arithmetic.VariablePrecisionDSPBlock', 'mult1_adder_available', 101);|alt_dspbuilder_update_gui('BlockFactory', 'com.altera.dspbuilder.blockset.arithmetic.VariablePrecisionDSPBlock', 'mult1_direction', 102);|alt_dspbuilder_update_gui('BlockFactory', 'com.altera.dspbuilder.blockset.arithmetic.VariablePrecisionDSPBlock', 'mult3_adder_available', 103);|alt_dspbuilder_update_gui('BlockFactory', 'com.altera.dspbuilder.blockset.arithmetic.VariablePrecisionDSPBlock', 'mult3_direction', 104);|alt_dspbuilder_update_gui('BlockFactory', 'com.altera.dspbuilder.blockset.arithmetic.VariablePrecisionDSPBlock', 'chainout_adder_available', 105);|alt_dspbuilder_update_gui('BlockFactory', 'com.altera.dspbuilder.blockset.arithmetic.VariablePrecisionDSPBlock', 'use_chainout_input', 106);|alt_dspbuilder_update_gui('BlockFactory', 'com.altera.dspbuilder.blockset.arithmetic.VariablePrecisionDSPBlock', 'chainout_input_used', 107);|alt_dspbuilder_update_gui('BlockFactory', 'com.altera.dspbuilder.blockset.arithmetic.VariablePrecisionDSPBlock', 'use_chainout_output', 108);|alt_dspbuilder_update_gui('BlockFactory', 'com.altera.dspbuilder.blockset.arithmetic.VariablePrecisionDSPBlock', 'chainout_output_used', 109);|alt_dspbuilder_update_gui('BlockFactory', 'com.altera.dspbuilder.blockset.arithmetic.VariablePrecisionDSPBlock', 'accum_available', 110);|alt_dspbuilder_update_gui('BlockFactory', 'com.altera.dspbuilder.blockset.arithmetic.VariablePrecisionDSPBlock', 'enable_accum', 111);|alt_dspbuilder_update_gui('BlockFactory', 'com.altera.dspbuilder.blockset.arithmetic.VariablePrecisionDSPBlock', 'accum_used', 112);|alt_dspbuilder_update_gui('BlockFactory', 'com.altera.dspbuilder.blockset.arithmetic.VariablePrecisionDSPBlock', 'double_accum_available', 113);|alt_dspbuilder_update_gui('BlockFactory', 'com.altera.dspbuilder.blockset.arithmetic.VariablePrecisionDSPBlock', 'enable_double_accum', 114);|alt_dspbuilder_update_gui('BlockFactory', 'com.altera.dspbuilder.blockset.arithmetic.VariablePrecisionDSPBlock', 'double_accum_used', 115);|alt_dspbuilder_update_gui('BlockFactory', 'com.altera.dspbuilder.blockset.arithmetic.VariablePrecisionDSPBlock', 'negate_available', 116);|alt_dspbuilder_update_gui('BlockFactory', 'com.altera.dspbuilder.blockset.arithmetic.VariablePrecisionDSPBlock', 'mult_add_operation', 117);|alt_dspbuilder_update_gui('BlockFactory', 'com.altera.dspbuilder.blockset.arithmetic.VariablePrecisionDSPBlock', 'rounding_constant_available', 118);|alt_dspbuilder_update_gui('BlockFactory', 'com.altera.dspbuilder.blockset.arithmetic.VariablePrecisionDSPBlock', 'use_rounding_constant', 119);|alt_dspbuilder_update_gui('BlockFactory', 'com.altera.dspbuilder.blockset.arithmetic.VariablePrecisionDSPBlock', 'rounding_constant_used', 120);||||||||||alt_dspbuilder_update_gui('BlockFactory', 'com.altera.dspbuilder.blockset.arithmetic.VariablePrecisionDSPBlock', 'reg_mult1_op_control', 130);|alt_dspbuilder_update_gui('BlockFactory', 'com.altera.dspbuilder.blockset.arithmetic.VariablePrecisionDSPBlock', 'enable_addnsub1_pipeline_reg', 131);||alt_dspbuilder_update_gui('BlockFactory', 'com.altera.dspbuilder.blockset.arithmetic.VariablePrecisionDSPBlock', 'reg_mult3_op_control', 133);|alt_dspbuilder_update_gui('BlockFactory', 'com.altera.dspbuilder.blockset.arithmetic.VariablePrecisionDSPBlock', 'reg_accum_control', 134);|alt_dspbuilder_update_gui('BlockFactory', 'com.altera.dspbuilder.blockset.arithmetic.VariablePrecisionDSPBlock', 'enable_accum_pipeline_reg', 135);||alt_dspbuilder_update_gui('BlockFactory', 'com.altera.dspbuilder.blockset.arithmetic.VariablePrecisionDSPBlock', 'reg_negate_control', 137);|alt_dspbuilder_update_gui('BlockFactory', 'com.altera.dspbuilder.blockset.arithmetic.VariablePrecisionDSPBlock', 'enable_negate_pipeline_reg', 138);|||alt_dspbuilder_update_gui('BlockFactory', 'com.altera.dspbuilder.blockset.arithmetic.VariablePrecisionDSPBlock', 'control_regs_ena', 141);|alt_dspbuilder_update_gui('BlockFactory', 'com.altera.dspbuilder.blockset.arithmetic.VariablePrecisionDSPBlock', 'control_pipeline_regs_ena', 142);|||
      mask TabNameString: Basic Structure,Basic Structure,Basic Structure,Basic Structure,Basic Structure,Basic Structure,Basic Structure,Basic Structure,Basic Structure,Basic Structure,Primary Data and Controls,Primary Data and Controls,Primary Data and Controls,Primary Data and Controls,Primary Data and Controls,Primary Data and Controls,Primary Data and Controls,Primary Data and Controls,Primary Data and Controls,Primary Data and Controls,Primary Data and Controls,Primary Data and Controls,Primary Data and Controls,Primary Data and Controls,Primary Data and Controls,Primary Data and Controls,Primary Data and Controls,Primary Data and Controls,Primary Data and Controls,Primary Data and Controls,Primary Data and Controls,Primary Data and Controls,Primary Data and Controls,Primary Data and Controls,Primary Data and Controls,Primary Data and Controls,Primary Data and Controls,Primary Data and Controls,Primary Data and Controls,Primary Data and Controls,Primary Data and Controls,Primary Data and Controls,Primary Data and Controls,Primary Data and Controls,Primary Data and Controls,Primary Data and Controls,Primary Data and Controls,Primary Data and Controls,Primary Data and Controls,Primary Data and Controls,Primary Data and Controls,Primary Data and Controls,Primary Data and Controls,Primary Data and Controls,Primary Data and Controls,Primary Data and Controls,Primary Data and Controls,Primary Data and Controls,Primary Data and Controls,Primary Data and Controls,Primary Data and Controls,Primary Data and Controls,Primary Data and Controls,Primary Data and Controls,Primary Data and Controls,Primary Data and Controls,Primary Data and Controls,Input Phase Structure,Input Phase Structure,Input Phase Structure,Input Phase Structure,Input Phase Structure,Input Phase Structure,Input Phase Structure,Input Phase Structure,Input Phase Structure,Input Phase Structure,Input Phase Structure,Input Phase Structure,Input Phase Structure,Input Phase Structure,Input Phase Structure,Input Phase Structure,Input Phase Structure,Input Phase Structure,Input Phase Structure,Input Phase Structure,Input Phase Structure,Input Phase Structure,Input Phase Structure,Input Phase Structure,Input Phase Structure,Input Phase Structure,Input Phase Structure,Input Phase Structure,Input Phase Structure,Input Phase Structure,Input Phase Structure,Input Phase Structure,Input Phase Structure,Input Phase Structure,Output Phase Structure,Output Phase Structure,Output Phase Structure,Output Phase Structure,Output Phase Structure,Output Phase Structure,Output Phase Structure,Output Phase Structure,Output Phase Structure,Output Phase Structure,Output Phase Structure,Output Phase Structure,Output Phase Structure,Output Phase Structure,Output Phase Structure,Output Phase Structure,Output Phase Structure,Output Phase Structure,Output Phase Structure,Output Phase Structure,Output Phase Structure,Optional Data and Control,Optional Data and Control,Optional Data and Control,Optional Data and Control,Optional Data and Control,Optional Data and Control,Optional Data and Control,Optional Data and Control,Optional Data and Control,Optional Data and Control,Optional Data and Control,Optional Data and Control,Optional Data and Control,Optional Data and Control,Optional Data and Control,Optional Data and Control,Optional Data and Control,Optional Data and Control,Optional Data and Control,Optional Data and Control,Optional Data and Control,Optional Data and Control,Optional Data and Control,Optional Data and Control
      mask Display:
      | port_label('input', 1, 'a0(7:0)');
      | port_label('input', 2, 'b0(7:0)');
      | port_label('output', 1, 'out(15:0)');
      | 
      | 
      | disp('out = a0 * b0');
  Virtual Pins : S-Function  LoadFcn=|  FunctionName=sTestBench  Parameters=enable  EnableBusSupport=off  mask(Virtual Pins AlteraBlockset){enable=on}
      | alt_dspbuilder_load_block(gcb, 'BlockFactory', 'com.altera.dspbuilder.blockset.altlab.VirtualPins');
      | alt_dspbuilder_init_virtualpins
      mask prompts: enable "Enable Virtual Pins"
      mask help: When enabled creates global assignments in the Quartus II project to force all the pins to be virtual.
      mask init:
      | alt_dspbuilder_init_virtualpins('BlockFactory', 'com.altera.dspbuilder.blockset.altlab.VirtualPins', { enable });
      settings: CopyFcn=alt_dspbuilder_add_block(gcb, 'BlockFactory', 'com.altera.dspbuilder.blockset.altlab.VirtualPins');  UndoDeleteFcn=alt_dspbuilder_add_block(gcb, 'BlockFactory', 'com.altera.dspbuilder.blockset.altlab.VirtualPins');  NameChangeFcn=alt_dspbuilder_block_renamed(gcb);
      settings: DeleteFcn=|
      | alt_dspbuilder_internal_remove_virtualpins(gcb)
      | 
      | com.altera.dspbuilder.simulation.Mask.delete(gcb);
      settings: PostSaveFcn=|
      | alt_dspbuilder_block_saved(gcb);
      | alt_dspbuilder_init_virtualpins
      mask Help: helpview(char(com.altera.dspbuilder.simulation.Cache.getBlockTemplate('BlockFactory', 'com.altera.dspbuilder.blockset.altlab.VirtualPins').getHelpFile))
      mask Display: fprintf('Virtual Pins\non');
